simulink model "New_density"  (Simulink 7.9)
settings: Solver=FixedStepDiscrete  StartTime=0.0  StopTime=0  FixedStep=1  RelTol=1e-3
undefined symbols (not defined in the file): Carnot_density_Callbacks
settings Model: DEBUGGLOBALLEVEL=1  DEBUGWRITETOFILE=0  DEBUGFILENAME=bla.txt  DEBUGMAXCONSECUTIVEWARNINGS=inf  DEBUGMAXTOTALWARNINGS=inf  Creator=awohlfei  LastModifiedBy=awohlfei

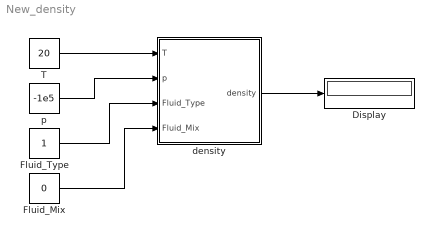
== system New_density ==
  Display : Display
  Fluid_Mix : Constant  Value=0
  Fluid_Type : Constant
  T : Constant  Value=20
  density : Subsystem  LoadFcn=Carnot_density_Callbacks('LoadFcn');  InitFcn=load('THB.mat');  VariantObject=CarlibClassic  mask(density){INPUTARGUMENTS=state variables (classic), DEBUGLEVEL=DEBUG, MAXTOTALWARNINGS=inf, MAXCONSECUTIVEWARNINGS=inf, WRITETOFILE=0, FILENAME='errors.txt'}
      mask prompts: INPUTARGUMENTS "Input arguments"; DEBUGLEVEL "Debug level"; MAXTOTALWARNINGS "maximum number of total warning"; MAXCONSECUTIVEWARNINGS "maximum number of consecutive warnings"; WRITETOFILE "write messages to file"; FILENAME "filename for error messages"
      mask help:
      | Calculates the fluid density  [kg/m³].
      | Calls the function "density" in the CARNOT library "carlib".
      mask init:
      | %Inports
      | Carnot_density_Callbacks('CreateInports');
      | 
      | %global debug level
      | [DEBUGLEVEL, MAXTOTALWARNINGS, MAXCONSECUTIVEWARNINGS, WRITETOFILE, FILENAME] = Carnot_density_Callbacks('CheckDebugLevels', DEBUGLEVEL, MAXTOTALWARNINGS, MAXCONSECUTIVEWARNINGS, WRITETOFILE, FILENAME);
      mask StyleString: popup(state variables (classic)|THB|THV),popup(DEBUG|INFO|WARNING|ERROR|FATAL|NONE),edit,edit,edit,edit
      mask CallbackString: Carnot_density_Callbacks('MaskVisibilities');|||||
      mask TabNameString: Parameters,Debugging,Debugging,Debugging,Debugging,Debugging
  p : Constant  Value=-1e5
  wires:
  T/1 -> density/1(T)
  p/1 -> density/2(p)
  Fluid_Type/1 -> density/3(Fluid_Type)
  Fluid_Mix/1 -> density/4(Fluid_Mix)
  density/1(density) -> Display/1

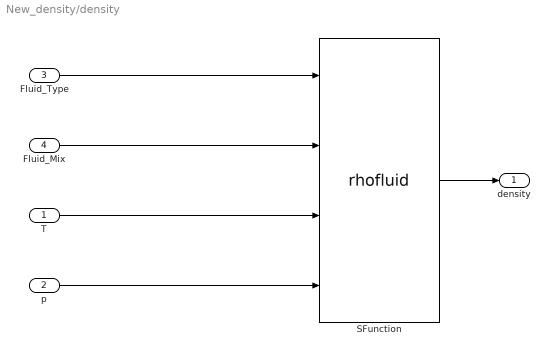
== system New_density/density ==
  T : Inport
  p : Inport  Port=2
  Fluid_Type : Inport  Port=3
  Fluid_Mix : Inport  Port=4
  SFunction : S-Function  FunctionName=rhofluid  Parameters=DEBUGLEVEL,MAXTOTALWARNINGS,MAXCONSECUTIVEWARNINGS,WRITETOFILE,FILENAME  EnableBusSupport=off
  density : Outport
  wires:
  SFunction/1 -> density/1
  T/1 -> SFunction/3
  p/1 -> SFunction/4
  Fluid_Type/1 -> SFunction/1
  Fluid_Mix/1 -> SFunction/2
